simulink model "midProj"  (R2021b)
settings: Solver=VariableStepAuto  StartTime=0.0  StopTime=8  RelTol=1e-3
values from neighbouring files (symbols this model uses):
  X = 1    [initialSim.m]
  Y = 1    [initialSim.m]
undefined symbols (not defined in the file or in its folder): Discrete, PhiDesire, PhoDesire, Time
libraries: simulink x2, slpidlib x2, ctrlSharedLib x1
settings Model: Creator=yuhaiyang  LastModifiedBy=yuhaiyang
settings SolverCC: AlgebraicLoopSolver=TrustRegion
settings DebuggingCC: SFMachineParentedDataDiag=warning

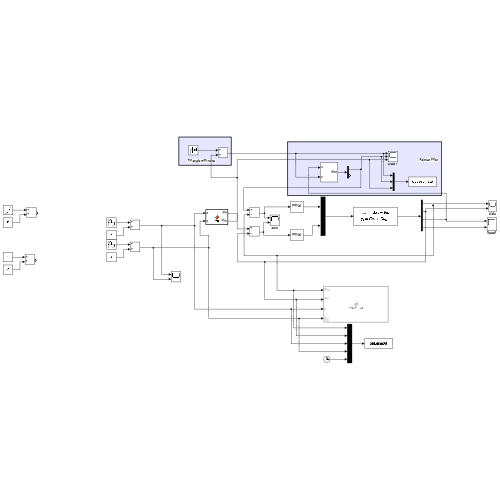
[thumbnail: Simulink's stored preview of the top-level diagram]
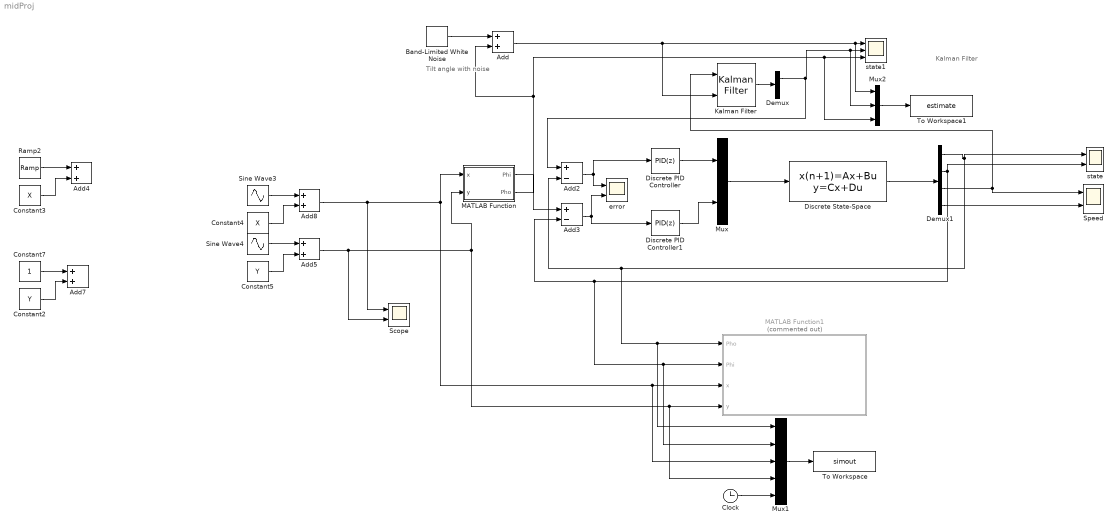
== system midProj ==
  note: Kalman Filter
  note: Tilt angle with noise
  Add{,4..5,7..8} (5 alike) : Sum
  Add2 : Sum  Inputs=+-
  Add3 : Sum  Inputs=+-
  Band-Limited White Noise : simulink/Sources/Band-Limited White Noise  Cov=[0.01]  Ts=0.05  seed=[23341]
  Clock : Clock
  Constant2 : Constant  Value=Y
  Constant3 : Constant  Value=X
  Constant4 : Constant  Value=X
  Constant5 : Constant  Value=Y
  Constant7 : Constant
  Demux : Demux  Outputs=2
  Demux1 : Demux
  Discrete PID Controller : slpidlib/PID Controller  Controller=PID  Form=Parallel  TimeDomain=Discrete-time  UseExternalTs=off  SampleTime=step  IntegratorMethod=Forward Euler  FilterMethod=Forward Euler  ControllerParametersSource=internal  P=0.0451594253248729  I=0.00606949033779435  D=0.0825217736897104  UseFilter=on  N=17.4747024685303  TunerSelectOption=Transfer Function Based (PID Tuner App)  InitialConditionSource=internal  InitialConditionForIntegrator=0  InitialConditionForFilter=0  DifferentiatorICPrevScaledInput=0  ExternalReset=none  TrackingMode=off  Kt=1  LimitOutput=off  SatLimitsSource=internal  UpperSaturationLimit=inf  LowerSaturationLimit=-inf  LinearizeAsGain=off  AntiWindupMode=none  Kb=1  POutMin=[]  POutMax=[]  IOutMin=[]  IOutMax=[]  DOutMin=[]  DOutMax=[]  NOutMin=[]  NOutMax=[]  SumOutMin=[]  SumOutMax=[]  SaturationOutMin=[]  SaturationOutMax=[]  PParamMin=[]  PParamMax=[]  IParamMin=[]  IParamMax=[]  DParamMin=[]  DParamMax=[]  NParamMin=[]  NParamMax=[]  KbParamMin=[]  KbParamMax=[]  KtParamMin=[]  KtParamMax=[]  KbOutMin=[]  KbOutMax=[]  KtOutMin=[]  KtOutMax=[]  IntegratorOutMin=[]  IntegratorOutMax=[]  FilterOutMin=[]  FilterOutMax=[]  SumI1OutMin=[]  SumI1OutMax=[]  SumI2OutMin=[]  SumI2OutMax=[]  SumI3OutMin=[]  SumI3OutMax=[]  SumI4OutMin=[]  SumI4OutMax=[]  SumDOutMin=[]  SumDOutMax=[]  DifferentiatorOutMin=[]  DifferentiatorOutMax=[]  FilterDiffOutCoefMin=[]  FilterDiffOutCoefMax=[]  ReciprocalOutMin=[]  ReciprocalOutMax=[]  SumDenOutMin=[]  SumDenOutMax=[]  SumNumOutMin=[]  SumNumOutMax=[]  DivideOutMin=[]  DivideOutMax=[]  UdiffTsProdOutMin=[]  UdiffTsProdOutMax=[]  NTsProdOutMin=[]  NTsProdOutMax=[]  UintegralTsProdOutMin=[]  UintegralTsProdOutMax=[]  UngainTsProdOutMin=[]  UngainTsProdOutMax=[]  IntegratorContinuousStateAttributes=''  IntegratorStateMustResolveToSignalObject=off  IntegratorRTWStateStorageClass=Auto  FilterContinuousStateAttributes=''  FilterStateMustResolveToSignalObject=off  FilterRTWStateStorageClass=Auto  ParallelPVariant=InternalParameters  IdealPVariant=Disabled  IVariant=InternalParameters  DVariant=InternalParameters  IntegratorVariant=Discrete  SatVariant=Disabled  AWVariant=Passthrough  PCopyVariant=Disabled  TRVariant=Disabled  FdbkBlocksVariant=Forward  IdealPFdbkVariant=Disabled  SatFdbkVariant=Disabled  DerivativeFilterVariant=ForwardEulerFilter  NVariant=InternalParameters  NCopyVariant=Disabled  FilterICVariant=InternalICsFilter  IntegratorICVariant=InternalICs  ExternalResetVariant=Disabled  TRSumVariant=Passthrough  SumFdbkVariant=Disabled  SumVariant=Sum_PID  TsampFilterVariant=InternalTs  TsampNgainVariant=Passthrough  TsampIntegralVariant=Passthrough  ExternalSaturationOutDataTypeStr=Inherit: Same as second input
  Discrete PID Controller1 : slpidlib/PID Controller  Controller=PID  Form=Parallel  TimeDomain=Discrete-time  UseExternalTs=off  SampleTime=step  IntegratorMethod=Forward Euler  FilterMethod=Forward Euler  ControllerParametersSource=internal  P=0.0143220434066502  I=0.00109223482739123  D=0.0463013739503765  UseFilter=on  N=12.1025626011462  TunerSelectOption=Transfer Function Based (PID Tuner App)  InitialConditionSource=internal  InitialConditionForIntegrator=0  InitialConditionForFilter=0  DifferentiatorICPrevScaledInput=0  ExternalReset=none  TrackingMode=off  Kt=1  LimitOutput=off  SatLimitsSource=internal  UpperSaturationLimit=inf  LowerSaturationLimit=-inf  LinearizeAsGain=off  AntiWindupMode=none  Kb=1  POutMin=[]  POutMax=[]  IOutMin=[]  IOutMax=[]  DOutMin=[]  DOutMax=[]  NOutMin=[]  NOutMax=[]  SumOutMin=[]  SumOutMax=[]  SaturationOutMin=[]  SaturationOutMax=[]  PParamMin=[]  PParamMax=[]  IParamMin=[]  IParamMax=[]  DParamMin=[]  DParamMax=[]  NParamMin=[]  NParamMax=[]  KbParamMin=[]  KbParamMax=[]  KtParamMin=[]  KtParamMax=[]  KbOutMin=[]  KbOutMax=[]  KtOutMin=[]  KtOutMax=[]  IntegratorOutMin=[]  IntegratorOutMax=[]  FilterOutMin=[]  FilterOutMax=[]  SumI1OutMin=[]  SumI1OutMax=[]  SumI2OutMin=[]  SumI2OutMax=[]  SumI3OutMin=[]  SumI3OutMax=[]  SumI4OutMin=[]  SumI4OutMax=[]  SumDOutMin=[]  SumDOutMax=[]  DifferentiatorOutMin=[]  DifferentiatorOutMax=[]  FilterDiffOutCoefMin=[]  FilterDiffOutCoefMax=[]  ReciprocalOutMin=[]  ReciprocalOutMax=[]  SumDenOutMin=[]  SumDenOutMax=[]  SumNumOutMin=[]  SumNumOutMax=[]  DivideOutMin=[]  DivideOutMax=[]  UdiffTsProdOutMin=[]  UdiffTsProdOutMax=[]  NTsProdOutMin=[]  NTsProdOutMax=[]  UintegralTsProdOutMin=[]  UintegralTsProdOutMax=[]  UngainTsProdOutMin=[]  UngainTsProdOutMax=[]  IntegratorContinuousStateAttributes=''  IntegratorStateMustResolveToSignalObject=off  IntegratorRTWStateStorageClass=Auto  FilterContinuousStateAttributes=''  FilterStateMustResolveToSignalObject=off  FilterRTWStateStorageClass=Auto  ParallelPVariant=InternalParameters  IdealPVariant=Disabled  IVariant=InternalParameters  DVariant=InternalParameters  IntegratorVariant=Discrete  SatVariant=Disabled  AWVariant=Passthrough  PCopyVariant=Disabled  TRVariant=Disabled  FdbkBlocksVariant=Forward  IdealPFdbkVariant=Disabled  SatFdbkVariant=Disabled  DerivativeFilterVariant=ForwardEulerFilter  NVariant=InternalParameters  NCopyVariant=Disabled  FilterICVariant=InternalICsFilter  IntegratorICVariant=InternalICs  ExternalResetVariant=Disabled  TRSumVariant=Passthrough  SumFdbkVariant=Disabled  SumVariant=Sum_PID  TsampFilterVariant=InternalTs  TsampNgainVariant=Passthrough  TsampIntegralVariant=Passthrough  ExternalSaturationOutDataTypeStr=Inherit: Same as second input
  Discrete State-Space : DiscreteStateSpace  A=|  B=|  C=[1,0,0,0;0,1,0,0;0,0,1,0;0,0,0,1]  D=[0,0;0,0;0,0;0,0]  InitialCondition=[PhoDesire,PhiDesire,0,0]'  SampleTime=step
      A=|
      | [1,0,step,0;
      |     0,1,0,step;
      |     0,0,1,0;
      |     0,0,0,1];
      B=|
      | [0,0;
      |     0,0;
      |     100*pi/180,0;
      |     0,100*pi/180];
  Kalman Filter : ctrlSharedLib/Kalman Filter  TimeDomain=Discrete-Time  UseCurrentEstimator=on  ModelSource=Individual A, B, C, D matrices  ModelSourceVariable=ss(0.95,1,1,0,1)  A=[1, step; 0,0]  B=[0;1]  C=[1,0]  D=0  NumberOfStates=1  NumberOfInputs=1  NumberOfOutputs=1  InitialEstimateSource=Dialog  X0=[pi,0]  P0=10  UseK=off  UseGH=off  NumberOfProcessNoiseInputs=1  G=1  TimeInvariantG=on  H=0  TimeInvariantH=on  Q=0.005  TimeInvariantQ=on  R=2  TimeInvariantR=on  N=0  TimeInvariantN=on  AddInputPort=on  AddEnablePort=off  OutputEstimatedY=off  OutputP=off  Ts=-1
  MATLAB Function : MATLAB Function  TreatAsAtomicUnit=on
  MATLAB Function1 : MATLAB Function  Commented=on  TreatAsAtomicUnit=on
  Mux : Mux  Inputs=2
  Mux1 : Mux  Inputs=5
  Mux2 : Mux  Inputs=3
  Ramp2 : simulink/Sources/Ramp  slope=0.2  start=0  InitialOutput=0
  Scope : Scope  NumInputPorts=2
  Sine Wave3 : Sin  Frequency=0.5  SampleTime=step
  Sine Wave4 : Sin  Frequency=0.5  Phase=pi/2  SampleTime=step
  Speed : Scope  NumInputPorts=2
  To Workspace : ToWorkspace  VariableName=simout  SampleTime=-1
      settings: Save2DSignal=2-D array (concatenate along first dimension)
  To Workspace1 : ToWorkspace  VariableName=estimate  SampleTime=-1
      settings: Save2DSignal=2-D array (concatenate along first dimension)
  "error " : Scope  NumInputPorts=2
  state : Scope  NumInputPorts=2
  state1 : Scope  NumInputPorts=3
  wires:
  Mux/1 -> Discrete State-Space/1
  Discrete State-Space/1 -> Demux1/1
  Demux1/1 -> state/1, Add2/2, Mux1/1, MATLAB Function1/1(Pho)
  Demux1/2 -> Mux1/2, MATLAB Function1/2(Phi), Add3/2, state/2
  Add2/1 -> Discrete PID Controller/1, "error "/1
  Add3/1 -> "error "/2, Discrete PID Controller1/1
  Discrete PID Controller/1 -> Mux/1
  Discrete PID Controller1/1 -> Mux/2
  Add5/1 -> Scope/2, MATLAB Function/2(y), Mux1/4, MATLAB Function1/4(y)
  MATLAB Function/2(Pho) -> Mux2/3, state1/3, Add/2
  MATLAB Function/1(Phi) -> Add3/1
  Add8/1 -> Scope/1, MATLAB Function/1(x), Mux1/3, MATLAB Function1/3(x)
  Mux1/1 -> To Workspace/1
  Clock/1 -> Mux1/5
  Ramp2/1 -> Add4/1
  Constant3/1 -> Add4/2
  Kalman Filter/1 -> Demux/1
  Demux1/4 -> Speed/2
  Add/1 -> Kalman Filter/2, Mux2/1, state1/1
  Demux1/3 -> Kalman Filter/1, Speed/1
  Demux/1 -> Add2/1, Mux2/2, state1/2
  Band-Limited White Noise/1 -> Add/1
  Constant2/1 -> Add7/2
  Constant7/1 -> Add7/1
  Mux2/1 -> To Workspace1/1
  Sine Wave4/1 -> Add5/1
  Constant5/1 -> Add5/2
  Constant4/1 -> Add8/2
  Sine Wave3/1 -> Add8/1

== matlab function midProj/MATLAB Function1 ==
  data: Pho input; Phi input; x input; y input
function detectPlot(Pho,Phi,x,y)

X = 1;
Y = 1;
Z = 6;
z = 0;
axis([-1 3 -1 3,0,6])
detect(X,Y,Z,Pho,Phi);
alpha(0.25);
hold on
plot3(x,y,z,'r*')
hold on

== matlab function midProj/MATLAB Function ==
  data: x input; Phi output; y input; Pho output
function [Phi,Pho] = fcn(x,y)
z = 0;
X = 1;
Y = 1;
Z = 6;

dist = sqrt((x-X)^2+(y-Y)^2+(z-Z)^2);
Phi = acos((z-Z)/dist);

if y<Y
    Pho = atan(-(x-X)/(y-Y));
elseif y>Y
    Pho = pi+atan(-(x-X)/(y-Y));
else
    if x>X
        Pho = pi/2;
    else
        Pho = pi+pi/2;
    end
end
